simulink model "sltestThrottlePositionControlCompositionExample"  (R2023a)
settings: Solver=FixedStepDiscrete  StartTime=0.0  StopTime=1.5  FixedStep=0.005  RelTol=1e-3  EnableMultiTasking=on
undefined symbols (not defined in the file or in its folder): D1, P
settings Model: Creator=The MathWorks, Inc.  LastModifiedBy=The MathWorks, Inc.
settings SolverCC: AlgebraicLoopSolver=TrustRegion  AutoInsertRateTranBlk=on  MaxZcPerStep=1
settings DataIOCC: SaveFormat=StructureWithTime  ReturnWorkspaceOutputs=off
settings OptimizationCC: DefaultParameterBehavior=Inlined  PassReuseOutputArgsAs=Individual arguments  ZeroExternalMemoryAtStartup=off  ZeroInternalMemoryAtStartup=off  EfficientTunableParamExpr=on
settings DebuggingCC: ParameterTunabilityLossMsg=error  UnconnectedInputMsg=warning  UnconnectedOutputMsg=warning  UnconnectedLineMsg=warning  PregeneratedLibrarySubsystemCodeDiagnostic=none  ArithmeticOperatorsInVariantConditions=warning
settings ModelReferenceCC: ModelReferenceNumInstancesAllowed=Single
settings SFSimCC: SimUseLocalCustomCode=off  MATLABDynamicMemAlloc=off  CustomCodeUndefinedFunction=UseInterfaceOnly
settings RTWCC: Description=AUTOSAR  SystemTargetFile=autosar.tlc  GenCodeOnly=on  TemplateMakefile=ert_default_tmf  GenerateReport=on  RTWUseLocalCustomCode=off  IncludeHyperlinkInReport=on  LaunchReport=on  PortableWordSizes=on  GenerateTraceInfo=on  GenerateTraceReport=on  GenerateTraceReportSl=on  GenerateTraceReportSf=on  GenerateTraceReportEml=on  DLArmComputeVersion=19.05
settings CodeAppCC: ForceParamTrailComments=on  IgnoreCustomStorageClasses=off  OperatorAnnotations=on  SimulinkDataObjDesc=on  SFDataObjDesc=on  InsertBlockDesc=on
settings STFCustomTargetCC: MultiwordLength=256  ParMdlRefBuildCompliant=on  CompOptLevelCompliant=on  ConcurrentExecutionCompliant=off  IncludeMdlTerminateFcn=off  CombineOutputUpdateFcns=on  SuppressErrorStatus=on  ERTCustomFileBanners=on  SupportNonFinite=off  SupportComplex=off  SupportContinuousTime=off  SupportNonInlinedSFcns=off  RemoveResetFunc=on  MATLABClassNameForMDSCustomization=Simulink.SoftwareTarget.ERTCustomization  CPPClassGenCompliant=on  AutosarCompliant=on  GRTInterface=off  LookupTableObjectStructAxisOrder=2,1,3,4,...  LUTObjectStructOrderEvenSpacing=Size,Table,Breakpoints  SystemTargetFile=autosar.tlc
settings ERTTargetCC: TargetLangStandard=C99 (ISO)  ConcurrentExecutionCompliant=off  IncludeMdlTerminateFcn=off  SuppressErrorStatus=on  SupportNonFinite=off  SupportComplex=off  ModelStepFunctionPrototypeControlCompliant=off  AutosarCompliant=on  LookupTableObjectStructAxisOrder=2,1,3,4,...  LUTObjectStructOrderEvenSpacing=Size,Table,Breakpoints  InlinedParameterPlacement=NonHierarchical  ERTCustomFileTemplate=example_file_process.tlc

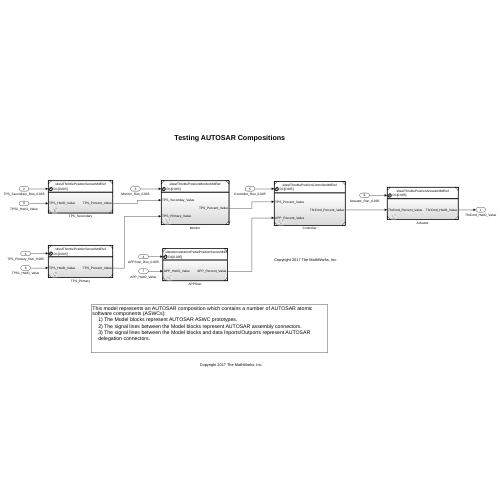
[thumbnail: Simulink's stored preview of the top-level diagram]
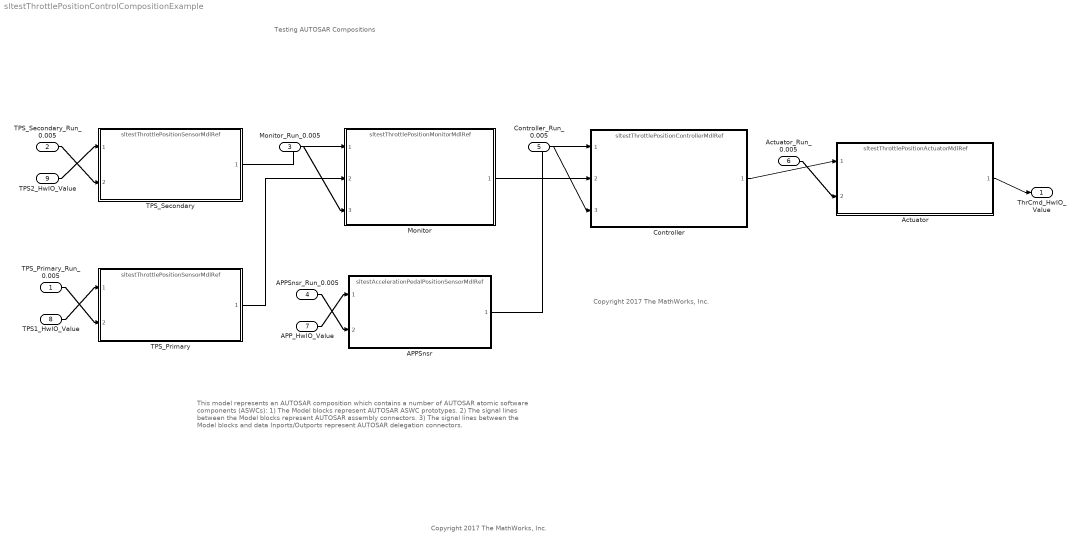
== system sltestThrottlePositionControlCompositionExample ==
  note: Copyright 2017 The MathWorks, Inc.
  note: Testing AUTOSAR Compositions
  note: This model represents an AUTOSAR composition which contains a number of AUTOSAR atomic software components (ASWCs):
      | 1) The Model blocks represent AUTOSAR ASWC prototypes.
      | 2) The signal lines between the Model blocks represent AUTOSAR assembly connectors.
      | 3) The signal lines between the Model blocks and data Inports/Outports represent AUTOSAR delegation connectors.
  note: Copyright 2017 The MathWorks, Inc.
  TPS_Primary_Run_0.005 : Inport  SampleTime=0.005  OutputFunctionCall=on
  TPS_Secondary_Run_0.005 : Inport  Port=2  SampleTime=0.005  OutputFunctionCall=on
  Monitor_Run_0.005 : Inport  Port=3  SampleTime=0.005  OutputFunctionCall=on
  APPSnsr_Run_0.005 : Inport  Port=4  SampleTime=0.005  OutputFunctionCall=on
  Controller_Run_0.005 : Inport  Port=5  SampleTime=0.005  OutputFunctionCall=on
  Actuator_Run_0.005 : Inport  Port=6  SampleTime=0.005  OutputFunctionCall=on
  APP_HwIO_Value : Inport  Port=7  OutDataTypeStr=uint16  PortDimensions=1
  TPS1_HwIO_Value : Inport  Port=8  OutDataTypeStr=uint16  PortDimensions=1
  TPS2_HwIO_Value : Inport  Port=9  OutDataTypeStr=uint16  PortDimensions=1
  APPSnsr : ModelReference  ModelNameDialog=sltestAccelerationPedalPositionSensorMdlRef  SimulationMode=Normal  ScheduleRates=on  PortDiscreteRates=0.005  CachedPortDiscreteRates=[0.005]  ModelEventPortInfo=P:D1[0.005][0][0]  ModelReferenceVersion=4.0
  Actuator : ModelReference  ModelNameDialog=sltestThrottlePositionActuatorMdlRef  SimulationMode=Normal  ScheduleRates=on  PortDiscreteRates=0.005  CachedPortDiscreteRates=[0.005]  ModelEventPortInfo=P:D1[0.005][0][0]  ModelReferenceVersion=4.0
  Controller : ModelReference  ModelNameDialog=sltestThrottlePositionControllerMdlRef  SimulationMode=Normal  ScheduleRates=on  PortDiscreteRates=0.005  CachedPortDiscreteRates=[0.005]  ModelEventPortInfo=P:D1[0.005][0][0]  CodeInterface=Top model  ModelReferenceVersion=4.0
  Monitor : ModelReference  ModelNameDialog=sltestThrottlePositionMonitorMdlRef  SimulationMode=Normal  ScheduleRates=on  PortDiscreteRates=0.005  CachedPortDiscreteRates=[0.005]  ModelEventPortInfo=P:D1[0.005][0][0]  CodeInterface=Top model  ModelReferenceVersion=4.0
  TPS_Primary : ModelReference  ModelNameDialog=sltestThrottlePositionSensorMdlRef  SimulationMode=Normal  ScheduleRates=on  PortDiscreteRates=0.005  CachedPortDiscreteRates=[0.005]  ModelEventPortInfo=P:D1[0.005][0][0]  ModelReferenceVersion=4.0
  TPS_Secondary : ModelReference  ModelNameDialog=sltestThrottlePositionSensorMdlRef  SimulationMode=Normal  ScheduleRates=on  PortDiscreteRates=0.005  CachedPortDiscreteRates=[0.005]  ModelEventPortInfo=P:D1[0.005][0][0]  ModelReferenceVersion=4.0
  ThrCmd_HwIO_Value : Outport  OutDataTypeStr=int16  PortDimensions=1  VectorParamsAs1DForOutWhenUnconnected=off
  wires:
  APPSnsr/1 -> Controller/2
  Controller/1 -> Actuator/1
  Monitor/1 -> Controller/1
  TPS_Primary/1 -> Monitor/2
  TPS_Secondary/1 -> Monitor/1
  APP_HwIO_Value/1 -> APPSnsr/1
  APPSnsr_Run_0.005/1 -> APPSnsr/2
  Actuator_Run_0.005/1 -> Actuator/2
  Actuator/1 -> ThrCmd_HwIO_Value/1
  Controller_Run_0.005/1 -> Controller/3
  Monitor_Run_0.005/1 -> Monitor/3
  TPS_Primary_Run_0.005/1 -> TPS_Primary/2
  TPS2_HwIO_Value/1 -> TPS_Secondary/1
  TPS_Secondary_Run_0.005/1 -> TPS_Secondary/2
  TPS1_HwIO_Value/1 -> TPS_Primary/1
